simulink model "zustandsregler_simulink"  (R2025a)
settings: Solver=VariableStepAuto  StartTime=0.0  StopTime=20  RelTol=1e-3
values from neighbouring files (symbols this model uses):
  A = [0 1 0 0 ... (first row only)    [reglerInit.m]    (also in test_init.m; zustandsregler.m)
  B = [0; -30.49; 0; 30.49]    [reglerInit.m]    (also in test_init.m; zustandsregler.m)
  C_new = [1 0 0 0 ... (first row only)    [reglerInit.m]    (also in test_init.m; zustandsregler.m)
  K = place(A,B,pole)    [zustandsregler.m]
  v = -1/(C_vorfilter*(inv(A-B*K)*B))    [zustandsregler.m]
  x0 = [0; 0; 1; 0]    [reglerInit.m]    (also in test_init.m = [0; 0; 0; 0]; zustandsregler.m)
  zhut0 = [0;0;0;0]    [reglerInit.m]    (also in test_init.m; zustandsregler.m)
settings Model: Creator=marin  LastModifiedBy=marin

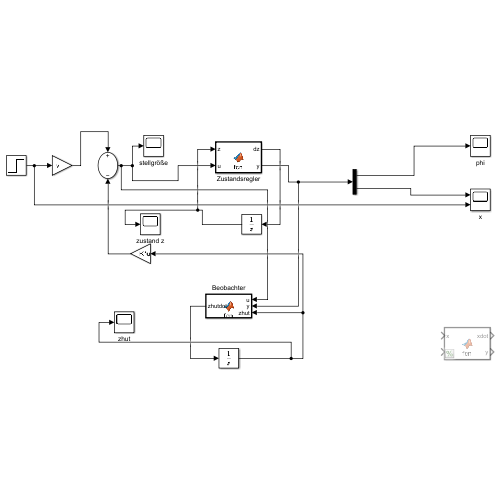
[thumbnail: Simulink's stored preview of the top-level diagram]
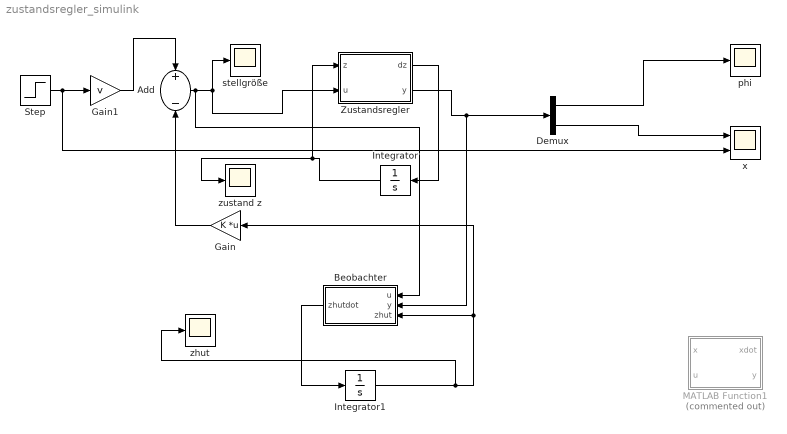
== system zustandsregler_simulink ==
  Add : Sum  Inputs=+-
  Beobachter : MATLAB Function  TreatAsAtomicUnit=on
  Demux : Demux  Outputs=2
  Gain : Gain  Gain=K  Multiplication=Matrix(K*u)
  Gain1 : Gain  Gain=v
  Integrator : Integrator  InitialCondition=x0
  Integrator1 : Integrator  InitialCondition=zhut0
  MATLAB Function1 : MATLAB Function  Commented=on  TreatAsAtomicUnit=on
  Step : Step  After=0.1  SampleTime=0
  Zustandsregler : MATLAB Function  TreatAsAtomicUnit=on
  phi : Scope
      settings: ActiveDisplayYMinimum=-0.34703471562841881  ActiveDisplayYMaximum=0.66563635310072589
  stellgröße : Scope
      settings: ActiveDisplayYMinimum=-0.47708072991756517  ActiveDisplayYMaximum=0.64386857946507492  DataLoggingVariableName=ScopeData4
  x : Scope  NumInputPorts=2
      settings: ActiveDisplayYMinimum=-0.93031960398854618  ActiveDisplayYMaximum=2.8583200864729181  DataLoggingVariableName=ScopeData2
  zhut : Scope
      settings: ActiveDisplayYMinimum=-1  ActiveDisplayYMaximum=1
  zustand z : Scope
      settings: ActiveDisplayYMinimum=-1  ActiveDisplayYMaximum=1  DataLoggingVariableName=ScopeData3
  wires:
  Zustandsregler/1(dz) -> Integrator/1
  Integrator/1 -> Zustandsregler/1(z), zustand z/1
  Demux/1 -> phi/1
  Demux/2 -> x/1
  Gain/1 -> Add/2
  Step/1 -> x/2, Gain1/1
  Gain1/1 -> Add/1
  Zustandsregler/2(y) -> Beobachter/2(y), Demux/1
  Integrator1/1 -> zhut/1, Gain/1, Beobachter/3(zhut)
  Add/1 -> Beobachter/1(u), Zustandsregler/2(u), stellgröße/1
  Beobachter/1(zhutdot) -> Integrator1/1

== matlab function zustandsregler_simulink/Zustandsregler ==
  data: z input; dz output; u input; y output
function [dz, y] = fcn(z, u)
    
    % Parameter
    l = 1;
    m_1 = 1;
    m_s = 0.8;
    r = 0.041;
    g = 9.81;
    k_r = 7.2e-3;
    
    % Zustände extrahieren (zur besseren Lesbarkeit)
    z1 = z(1);
    z2 = z(2);
    z3 = z(3);
    z4 = z(4);
    
    % Nenner-Term
    N = -m_1*cos(z1)^2 + m_1 + m_s; 
    
    % Nichtlinearer Zustandsvektor dz/dt = f(z,u)
    dz = zeros(4,1); 
    
    dz(1) = z2;
    dz(2) = -(l*m_1*r*cos(z1)*sin(z1)*z2^2 + u*cos(z1) + g*m_1*r*sin(z1) + g*m_s*r*sin(z1) - k_r*r*z4*cos(z1)) / (l*r*N);
    dz(3) = z4;
    dz(4) =  (l*m_1*r*sin(z1)*z2^2 + u - k_r*r*z4 + g*m_1*r*cos(z1)*sin(z1)) / (r*N);
    

    y = [z1; z3];

== matlab function zustandsregler_simulink/Beobachter ==
  data: u input; zhutdot output; y input; zhut input; A parameter; B parameter; C_new parameter; E parameter
function zhutdot = fcn(u, y, zhut, A, B, C_new, E)

zhutdot = (A-E*C_new)*zhut +B*u+E*y;

== matlab function zustandsregler_simulink/MATLAB Function1 ==
  data: x input; u input; xdot output; y output; B parameter; A parameter; C_new parameter
function [xdot,y] = fcn(x, u, B, A, C_new)

xdot= A*x+B*u;

y = C_new*x;
